simulink model "wangEx"  (R2014a)
settings: Solver=ode45  StartTime=0.0  StopTime=10.0  RelTol=1e-3
undefined symbols (not defined in the file): B, F, H, K, T
settings Model: Creator=sqn4594  LastModifiedBy=sqn4594

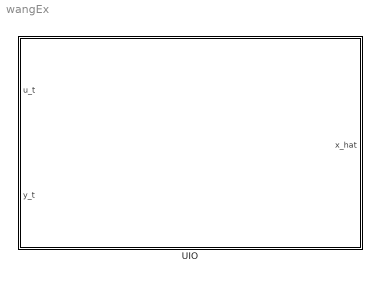
== system wangEx ==
  UIO : Subsystem

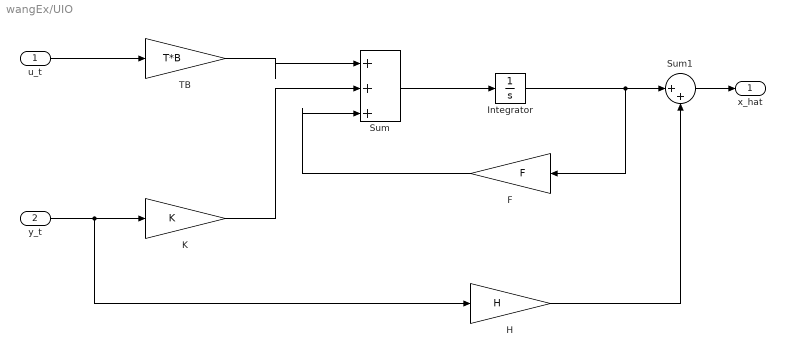
== system wangEx/UIO ==
  u_t : Inport
  y_t : Inport  Port=2
  F : Gain  Gain=F
  H : Gain  Gain=H
  Integrator : Integrator
  K : Gain  Gain=K
  Sum : Sum  Inputs=|+++
  Sum1 : Sum  Inputs=|++
  TB : Gain  Gain=T*B
  x_hat : Outport
  wires:
  u_t/1 -> TB/1
  y_t/1 -> H/1, K/1
  TB/1 -> Sum/1
  K/1 -> Sum/2
  Sum/1 -> Integrator/1
  Integrator/1 -> Sum1/1, F/1
  F/1 -> Sum/3
  H/1 -> Sum1/2
  Sum1/1 -> x_hat/1
